simulink model "gmsk_sync"  (Simulink 7.9)
settings: Solver=FixedStepDiscrete  SolverMode=SingleTasking  StartTime=0.0  StopTime=10.0  RelTol=1e-3
undefined symbols (not defined in the file or in its folder): addr, sync_pattern
libraries: shlslibv1 x45
settings Model: synDspstartup=OK  Creator=sszilvasi  LastModifiedBy=sszilvasi
settings DataIOCC: SaveOutput=off  SignalLogging=off  SaveTime=off
settings OptimizationCC: InlineParams=on
settings DebuggingCC: AlgebraicLoopMsg=error  InheritedTsInSrcMsg=none

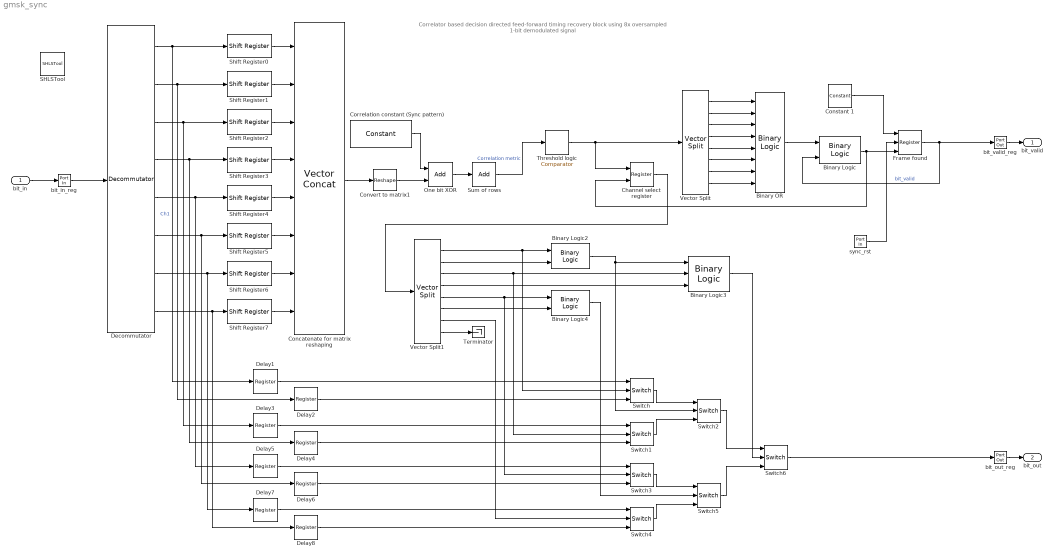
== system gmsk_sync ==
  note: Correlator based decision directed feed-forward timing recovery block
      | using 8x oversampled 1-bit demodulated signal
  bit_in : Inport
  Binary Logic : shlslibv1/Math Functions/Binary Logic  syn_binlog_exp=a&~b  synBlockType=primitive  synLatency=0  synBlockId=13
  Binary Logic2 : shlslibv1/Math Functions/Binary Logic  syn_binlog_exp=a|b  synBlockType=primitive  synLatency=0  synBlockId=13
  Binary Logic3 : shlslibv1/Math Functions/Binary Logic  syn_binlog_exp=a|b|c  synBlockType=primitive  synLatency=0  synBlockId=13
  Binary Logic4 : shlslibv1/Math Functions/Binary Logic  syn_binlog_exp=a|b  synBlockType=primitive  synLatency=0  synBlockId=13
  Binary OR : shlslibv1/Math Functions/Binary Logic  syn_binlog_exp=a|b|c|d|e|f|g|h  synBlockType=primitive  synLatency=0  synBlockId=13
  Channel select register : shlslibv1/Memories/Register  syn_delay_val=1  syn_rst_port=off  syn_en_port=on  synBlockType=custom  synLatency=1
  Concatenate for matrix reshaping : shlslibv1/Signal Operations/Vector Concat  syn_in_nb=8  syn_out_f=Full Precision  syn_out_wl=16  syn_out_fl=8  syn_out_dt=signed  synBlockType=primitive  synLatency=0  synBlockId=19
  Constant 1 : shlslibv1/Sources/Constant  syn_cst_val=1  syn_cst_fl=0  syn_cst_dt=unsigned  syn_cst_rnd=on  syn_cst_st=-1  synBlockType=primitive  synLatency=0  synBlockId=15
  Convert to matrix1 : shlslibv1/Signal Operations/Reshape  syn_op_dim_type=Specify  syn_op_dim=[length(sync_pattern) 8]  syn_ip_order=Row First  syn_op_order=Column First  syn_inh_port=off  synBlockType=primitive  synLatency=0  synBlockId=158
  Correlation constant (Sync pattern) : shlslibv1/Sources/Constant  syn_cst_val=fliplr(sync_pattern)'*ones(1,8)  syn_cst_fl=0  syn_cst_dt=unsigned  syn_cst_rnd=on  syn_cst_st=-1  synBlockType=primitive  synLatency=0  synBlockId=15
  Decommutator : shlslibv1/Signal Operations/Decommutator  syn_outport_nb=8  syn_outport_vec=off  synBlockType=custom  synLatency=1
  Delay{1..8} (8 alike) : shlslibv1/Memories/Register  syn_delay_val=1  syn_rst_port=off  syn_en_port=off  synBlockType=custom  synLatency=1
  Frame found : shlslibv1/Memories/Register  syn_delay_val=1  syn_rst_port=on  syn_en_port=on  synBlockType=custom  synLatency=1
  One bit XOR : shlslibv1/Math Functions/Add  syn_add_opr=++  syn_out_f=Specify  syn_out_wl=1  syn_out_fl=0  syn_out_dt=unsigned  syn_out_sat=off  syn_out_rnd=Floor (Truncate)  synBlockType=primitive  synLatency=0  synBlockId=96  syn_sum_of_rows=off
  SHLSTool : shlslibv1/SHLSTool  synBlockType=tool  syn_dsp_mode=FPGA
  Shift Register{0..7} (8 alike) : shlslibv1/Memories/Shift Register  syn_shift_dynamic=off  syn_shift_vec=[0:length(sync_pattern)-1]  syn_shift_val=16  syn_vect_out=Merge to vector  syn_rst_val=All zeros  syn_rst_vec=0  syn_rst_port=off  syn_en_port=off  synBlockType=primitive  synLatency=(addr+1)  synBlockId=93
  Sum of rows : shlslibv1/Math Functions/Add  syn_add_opr=+  syn_out_f=Specify  syn_out_wl=5  syn_out_fl=0  syn_out_dt=unsigned  syn_out_sat=off  syn_out_rnd=Floor (Truncate)  synBlockType=primitive  synLatency=0  synBlockId=96  syn_sum_of_rows=on
  Switch{,1..6} (7 alike) : shlslibv1/Signal Operations/Switch  switchCriteria=u2 > Threshold  switchThresh=0  synBlockType=custom  synLatency=0
  Terminator : Terminator
  Threshold logic : shlslibv1/Math Functions/Comparator  syn_comp_opr=a==b  syn_comp_const=on  syn_comp_val=0  synBlockType=primitive  synLatency=0  synBlockId=14
  Vector Split : shlslibv1/Signal Operations/Vector Split  syn_out_nb=8  synBlockType=primitive  synLatency=0  synBlockId=20
  Vector Split1 : shlslibv1/Signal Operations/Vector Split  syn_out_nb=8  synBlockType=primitive  synLatency=0  synBlockId=20
  bit_in_reg : shlslibv1/Ports & Subsystems/Port In  syn_out_wl=1  syn_out_fl=0  syn_out_dt=unsigned  syn_out_st=1  syn_capture=off  syn_register=on  syn_out_sat=off  syn_out_rnd=on  synBlockType=port  synLatency=1  synBlockId=0
  bit_out_reg : shlslibv1/Ports & Subsystems/Port Out  syn_capture=off  syn_register=on  synBlockType=port  synLatency=1  synBlockId=1
  bit_valid_reg : shlslibv1/Ports & Subsystems/Port Out  syn_capture=off  syn_register=on  synBlockType=port  synLatency=1  synBlockId=1
  sync_rst : shlslibv1/Ports & Subsystems/Port In  syn_out_wl=1  syn_out_fl=0  syn_out_dt=unsigned  syn_out_st=-1  syn_capture=off  syn_register=on  syn_out_sat=off  syn_out_rnd=off  synBlockType=port  synLatency=1  synBlockId=0
  bit_valid : Outport
  bit_out : Outport  Port=2
  wires:
  Decommutator/1 -> Shift Register0/1, Delay1/1  "Ch1"
  Decommutator/2 -> Shift Register1/1, Delay2/1
  Decommutator/3 -> Shift Register2/1, Delay3/1
  Decommutator/4 -> Shift Register3/1, Delay4/1
  Shift Register0/1 -> Concatenate for matrix reshaping/1
  Shift Register1/1 -> Concatenate for matrix reshaping/2
  Shift Register2/1 -> Concatenate for matrix reshaping/3
  Shift Register3/1 -> Concatenate for matrix reshaping/4
  Sum of rows/1 -> Threshold logic/1  "Correlation metric"
  One bit XOR/1 -> Sum of rows/1
  Concatenate for matrix reshaping/1 -> Convert to matrix1/1
  Vector Split/1 -> Binary OR/1
  Vector Split/2 -> Binary OR/2
  Vector Split/3 -> Binary OR/3
  Vector Split/4 -> Binary OR/4
  Switch/1 -> Switch2/1
  Switch1/1 -> Switch2/3
  Binary OR/1 -> Binary Logic/1
  Frame found/1 -> Binary Logic/2, bit_valid_reg/1  "bit_valid"
  Binary Logic/1 -> Frame found/3, Channel select register/2
  Constant 1/1 -> Frame found/1
  Vector Split1/1 -> Switch/2, Binary Logic2/1
  Vector Split1/3 -> Switch1/2, Binary Logic3/2
  Binary Logic2/1 -> Switch2/2, Binary Logic3/1
  Vector Split1/2 -> Binary Logic2/2
  Threshold logic/1 -> Vector Split/1, Channel select register/1
  Correlation constant (Sync pattern)/1 -> One bit XOR/1
  Decommutator/5 -> Shift Register4/1, Delay5/1
  Decommutator/6 -> Shift Register5/1, Delay6/1
  Decommutator/7 -> Shift Register6/1, Delay7/1
  Decommutator/8 -> Shift Register7/1, Delay8/1
  Shift Register4/1 -> Concatenate for matrix reshaping/5
  Shift Register5/1 -> Concatenate for matrix reshaping/6
  Shift Register6/1 -> Concatenate for matrix reshaping/7
  Shift Register7/1 -> Concatenate for matrix reshaping/8
  Vector Split/5 -> Binary OR/5
  Vector Split/6 -> Binary OR/6
  Vector Split/7 -> Binary OR/7
  Vector Split/8 -> Binary OR/8
  Switch3/1 -> Switch5/1
  Switch4/1 -> Switch5/3
  Switch5/1 -> Switch6/3
  Switch2/1 -> Switch6/1
  Switch6/1 -> bit_out_reg/1
  Vector Split1/5 -> Switch3/2, Binary Logic4/1
  Vector Split1/7 -> Switch4/2
  Vector Split1/6 -> Binary Logic4/2
  Binary Logic4/1 -> Switch5/2
  Vector Split1/4 -> Binary Logic3/3
  Binary Logic3/1 -> Switch6/2
  Convert to matrix1/1 -> One bit XOR/2
  bit_in_reg/1 -> Decommutator/1
  bit_in/1 -> bit_in_reg/1
  bit_valid_reg/1 -> bit_valid/1
  bit_out_reg/1 -> bit_out/1
  Vector Split1/8 -> Terminator/1
  Channel select register/1 -> Vector Split1/1
  Delay1/1 -> Switch/1
  Delay2/1 -> Switch/3
  Delay3/1 -> Switch1/1
  Delay4/1 -> Switch1/3
  Delay5/1 -> Switch3/1
  Delay6/1 -> Switch3/3
  Delay7/1 -> Switch4/1
  Delay8/1 -> Switch4/3
  sync_rst/1 -> Frame found/2
